simulink model "GNSS_Channel"  (R2025b)
settings: Solver=VariableStepAuto  StartTime=0.0  StopTime=599  RelTol=1e-3
libraries: commdigbbndpm3 x2, commchan3 x1
settings Model: Creator=heyia  LastModifiedBy=heyia

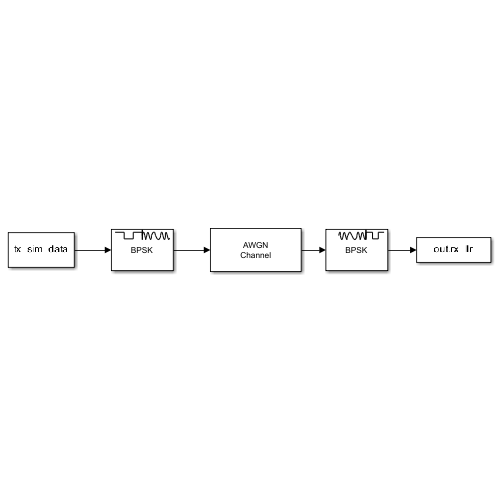
[thumbnail: Simulink's stored preview of the top-level diagram]
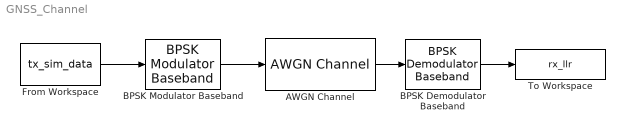
== system GNSS_Channel ==
  AWGN Channel : commchan3/AWGN Channel  LegacyMode=off  NoiseMethod="Signal to noise ratio  (SNR)"  noiseMode="Signal to noise ratio  (SNR)"  EbNo=10  EsNo=10  SNR=-1.5  BitsPerSymbol=1  SignalPower=1  SpecifySymbolPeriod=off  SamplesPerSymbol=1  SymbolPeriod=1  VarianceSource=Parameter  Variance=1  RandomStream=Global stream  Seed=67  SimulateUsing=Code generation
  BPSK Demodulator Baseband : commdigbbndpm3/BPSK Demodulator Baseband  DecType=Log-likelihood ratio  VarSource=Dialog  Variance=10^(1.5/10)  Ph=0  outDtype=Inherit via internal rule  derotateFactorWordLen=16  derotateFactorDataTypeStr=Inherit: Same word length as input  derotateFactorLastDataTypeStr=Inherit: Same word length as input
  BPSK Modulator Baseband : commdigbbndpm3/BPSK Modulator Baseband  Ph=0  outDtype=double  outWordLen=16  outUDDataType=sfix(16)  outFracLenMode=Best precision  outFracLen=15  outDataTypeStr=double  outLastDataTypeStr=double
  From Workspace : FromWorkspace  VariableName=tx_sim_data  SampleTime=1
  To Workspace : ToWorkspace  VariableName=rx_llr  SampleTime=-1
      settings: Save2DSignal=2-D array (concatenate along first dimension)
  wires:
  BPSK Modulator Baseband/1 -> AWGN Channel/1
  From Workspace/1 -> BPSK Modulator Baseband/1
  AWGN Channel/1 -> BPSK Demodulator Baseband/1
  BPSK Demodulator Baseband/1 -> To Workspace/1
